simulink library "PTOSim_Lib_Updated"  (R2020b)
settings: Solver=ode45  StartTime=0.0  StopTime=10.0  RelTol=1e-3  EnableMultiTasking=on
undefined symbols (not defined in the file or in its folder): DiscIntNeverNeededParam, pAeq, pAupper_limit, pBeq, pBupper_limit, ptosim, table
libraries: simulink x2, $bdroot x1
(part 2 of 2)

== system PTOSim_Lib_Updated/Generator/Direct Drive Rotary Generator/Subsystem ==
  vsdq : Inport
  wd : Inport  Port=2
  Add : Sum  Inputs=+-+
  Add1 : Sum  Inputs=--+
  Demux2 : Demux  Outputs=2
      settings: DisplayOption=none
  Fcn : Fcn  Expr=( u(1) - ptosim.lambda_fd ) / ptosim.Ls
  Gain : Gain  Gain=1/ptosim.Ls
  Gain1 : Gain  Gain=(pi*ptosim.radius/ptosim.tau_p)*ptosim.lambda_fd
  Gain2 : Gain  Gain=ptosim.Rs
  Gain3 : Gain  Gain=ptosim.Rs
  Integrator : Integrator  InitialCondition=ptosim.lambda_sd_0
  Integrator1 : Integrator  InitialCondition=ptosim.lambda_sq_0
  Mux : Mux  Inputs=2
  Product : Product  RndMeth=Zero
  Product1 : Product  RndMeth=Zero
  Tem : Outport
  isdq : Outport  Port=2
  wires:
  Add/1 -> Integrator/1  "d_dt_lambda_sd"
  Integrator/1 -> Product1/2, Fcn/1  "lambda_sd"
  Fcn/1 -> Gain3/1, Mux/1  "isd"
  Product/1 -> Add/1
  Add1/1 -> Integrator1/1  "d_dt_lambda_sq"
  Integrator1/1 -> Gain/1, Product/2  "lambda_sq"
  wd/1 -> Product1/1, Product/1
  Gain/1 -> Gain2/1, Mux/2, Gain1/1  "isq"
  Product1/1 -> Add1/1
  Demux2/1 -> Add/3  "vsd"
  Demux2/2 -> Add1/3  "vsq"
  vsdq/1 -> Demux2/1  "vsdq"
  Gain3/1 -> Add/2  "isd_Rs"
  Gain2/1 -> Add1/2
  Mux/1 -> isdq/1  "isdq"
  Gain1/1 -> Tem/1

== system PTOSim_Lib_Updated/Hydraulic/Compressible Fluid Piston/Pressure Bottom ==
  pos : Inport
  volFlowBottom : Inport  Port=2
  volFLowP : Inport  Port=3
  Constant1 : Constant  Value=ptosim.Vo
  Divide1 : Product  Inputs=*/
  Gain4 : Gain  Gain=ptosim.Beta_e
  Gain5 : Gain  Gain=ptosim.Ap
  Integrator3 : Integrator  InitialCondition=ptosim.pBi  UpperSaturationLimit=pBupper_limit  LowerSaturationLimit=pBeq
  Sum2 : Sum  Inputs=+-
  Sum3 : Sum
  bottomPressure : Outport
  wires:
  volFLowP/1 -> Sum2/2
  Integrator3/1 -> bottomPressure/1
  volFlowBottom/1 -> Sum2/1
  Divide1/1 -> Integrator3/1
  Sum3/1 -> Divide1/2
  Gain4/1 -> Divide1/1
  Constant1/1 -> Sum3/2
  Gain5/1 -> Sum3/1
  pos/1 -> Gain5/1
  Sum2/1 -> Gain4/1

== system PTOSim_Lib_Updated/Hydraulic/Compressible Fluid Piston/Pressure Top ==
  pos : Inport
  volFlowTop : Inport  Port=2
  volFlowP : Inport  Port=3
  Constant : Constant  Value=ptosim.Vo
  Divide : Product  Inputs=*/
  Gain1 : Gain  Gain=ptosim.Beta_e
  Gain2 : Gain  Gain=ptosim.Ap
  Integrator2 : Integrator  InitialCondition=ptosim.pAi  UpperSaturationLimit=pAupper_limit  LowerSaturationLimit=pAeq
  Sum : Sum
  Sum1 : Sum  Inputs=-+
  topPressure : Outport
  wires:
  volFlowP/1 -> Sum/2
  Integrator2/1 -> topPressure/1
  Divide/1 -> Integrator2/1
  volFlowTop/1 -> Sum/1
  Sum1/1 -> Divide/2
  Gain1/1 -> Divide/1
  Constant/1 -> Sum1/2
  Gain2/1 -> Sum1/1
  pos/1 -> Gain2/1
  Sum/1 -> Gain1/1

== system PTOSim_Lib_Updated/Hydraulic/Compressible Fluid Piston Updated/Subsystem ==
  Pos : Inport
  Vel : Inport  Port=2
  QB : Inport  Port=3
  Add : Sum
  Add1 : Sum  Inputs=--+
  Constant : Constant  Value=ptosim.Ap_B
  Constant1 : Constant  Value=ptosim.PistonStroke
  Constant2 : Constant  Value=ptosim.Ap_B
  Constant3 : Constant  Value=ptosim.BulkModulus
  Constant4 : Constant  Value=ptosim.xi_piston
  Divide : Product  Inputs=/*
  Product : Product
  Product1 : Product
  Product2 : Product
  Saturation : Saturate  UpperLimit=inf  LowerLimit=1e-12
  dPB_dt : Outport
  wires:
  Constant4/1 -> Add1/2
  Constant1/1 -> Add1/3
  Product1/1 -> dPB_dt/1
  Divide/1 -> Product1/1
  Constant3/1 -> Divide/2
  Product2/1 -> Saturation/1
  Constant2/1 -> Product2/2
  Add1/1 -> Product2/1
  Pos/1 -> Add1/1
  Add/1 -> Product1/2
  QB/1 -> Add/2
  Product/1 -> Add/1
  Constant/1 -> Product/2
  Vel/1 -> Product/1
  Saturation/1 -> Divide/1

== system PTOSim_Lib_Updated/Hydraulic/Compressible Fluid Piston Updated/dPa_dt ==
  Pos : Inport
  Vel : Inport  Port=2
  QA : Inport  Port=3
  Add : Sum  Inputs=-+
  Add1 : Sum
  Constant : Constant  Value=ptosim.Ap_A
  Constant1 : Constant  Value=ptosim.BulkModulus/ptosim.Ap_A
  Constant2 : Constant  Value=ptosim.xi_piston
  Divide : Product  Inputs=/*
  Product : Product
  Product1 : Product
  Saturation : Saturate  UpperLimit=inf  LowerLimit=1e-12
  dPA_dt : Outport
  wires:
  Constant2/1 -> Add1/1
  Add1/1 -> Saturation/1
  Pos/1 -> Add1/2
  Product/1 -> Add/1
  QA/1 -> Add/2
  Constant/1 -> Product/2
  Add/1 -> Product1/2
  Divide/1 -> dPA_dt/1
  Constant1/1 -> Product1/1
  Product1/1 -> Divide/2
  Vel/1 -> Product/1
  Saturation/1 -> Divide/1

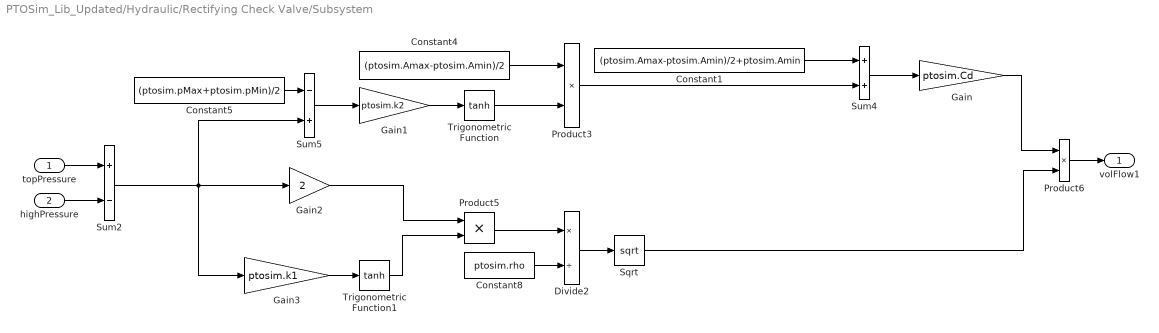
== system PTOSim_Lib_Updated/Hydraulic/Rectifying Check Valve/Subsystem ==
  topPressure : Inport
  highPressure : Inport  Port=2
  Constant1 : Constant  Value=(ptosim.Amax-ptosim.Amin)/2+ptosim.Amin
  Constant4 : Constant  Value=(ptosim.Amax-ptosim.Amin)/2
  Constant5 : Constant  Value=(ptosim.pMax+ptosim.pMin)/2
  Constant8 : Constant  Value=ptosim.rho
  Divide2 : Product  Inputs=*/
  Gain : Gain  Gain=ptosim.Cd
  Gain1 : Gain  Gain=ptosim.k2
  Gain2 : Gain  Gain=2
  Gain3 : Gain  Gain=ptosim.k1
  Product3 : Product
  Product5 : Product
  Product6 : Product
  Sqrt : Sqrt  SaturateOnIntegerOverflow=on
  Sum2 : Sum  Inputs=+-
  Sum4 : Sum
  Sum5 : Sum  Inputs=-+
  Trigonometric Function : Trigonometry  Operator=tanh
  Trigonometric Function1 : Trigonometry  Operator=tanh
  volFlow1 : Outport
  wires:
  Gain1/1 -> Trigonometric Function/1
  Trigonometric Function/1 -> Product3/2
  Product3/1 -> Sum4/2
  Sum5/1 -> Gain1/1
  Sum4/1 -> Gain/1
  Gain3/1 -> Trigonometric Function1/1
  Gain2/1 -> Product5/1
  Trigonometric Function1/1 -> Product5/2
  Sqrt/1 -> Product6/2
  Gain/1 -> Product6/1
  Constant8/1 -> Divide2/2
  Product5/1 -> Divide2/1
  Divide2/1 -> Sqrt/1
  topPressure/1 -> Sum2/1
  highPressure/1 -> Sum2/2
  Product6/1 -> volFlow1/1
  Constant4/1 -> Product3/1
  Constant5/1 -> Sum5/1
  Constant1/1 -> Sum4/1
  Sum2/1 -> Gain3/1, Sum5/2, Gain2/1

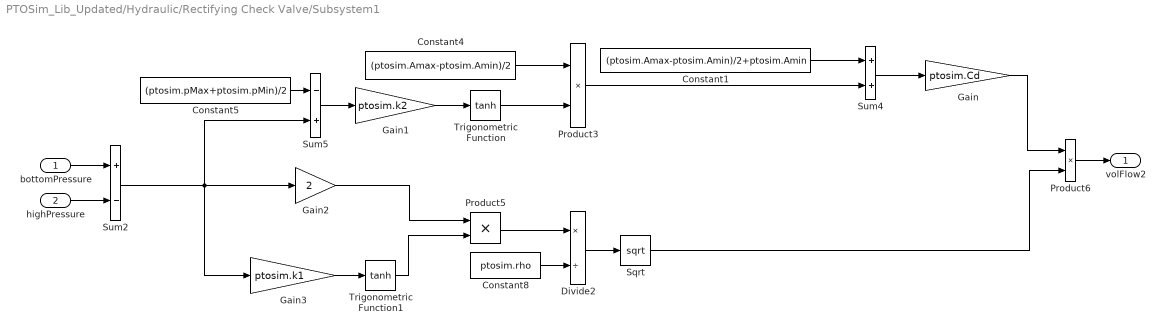
== system PTOSim_Lib_Updated/Hydraulic/Rectifying Check Valve/Subsystem1 ==
  bottomPressure : Inport
  highPressure : Inport  Port=2
  Constant1 : Constant  Value=(ptosim.Amax-ptosim.Amin)/2+ptosim.Amin
  Constant4 : Constant  Value=(ptosim.Amax-ptosim.Amin)/2
  Constant5 : Constant  Value=(ptosim.pMax+ptosim.pMin)/2
  Constant8 : Constant  Value=ptosim.rho
  Divide2 : Product  Inputs=*/
  Gain : Gain  Gain=ptosim.Cd
  Gain1 : Gain  Gain=ptosim.k2
  Gain2 : Gain  Gain=2
  Gain3 : Gain  Gain=ptosim.k1
  Product3 : Product
  Product5 : Product
  Product6 : Product
  Sqrt : Sqrt  SaturateOnIntegerOverflow=on
  Sum2 : Sum  Inputs=+-
  Sum4 : Sum
  Sum5 : Sum  Inputs=-+
  Trigonometric Function : Trigonometry  Operator=tanh
  Trigonometric Function1 : Trigonometry  Operator=tanh
  volFlow2 : Outport
  wires:
  Gain1/1 -> Trigonometric Function/1
  Trigonometric Function/1 -> Product3/2
  Product3/1 -> Sum4/2
  Sum5/1 -> Gain1/1
  Sum4/1 -> Gain/1
  Gain3/1 -> Trigonometric Function1/1
  Gain2/1 -> Product5/1
  Trigonometric Function1/1 -> Product5/2
  Sqrt/1 -> Product6/2
  Gain/1 -> Product6/1
  Constant8/1 -> Divide2/2
  Product5/1 -> Divide2/1
  Divide2/1 -> Sqrt/1
  bottomPressure/1 -> Sum2/1
  highPressure/1 -> Sum2/2
  Product6/1 -> volFlow2/1
  Constant4/1 -> Product3/1
  Constant5/1 -> Sum5/1
  Constant1/1 -> Sum4/1
  Sum2/1 -> Gain3/1, Sum5/2, Gain2/1

== system PTOSim_Lib_Updated/Hydraulic/Rectifying Check Valve/Subsystem2 ==
  lowPressure : Inport
  bottomPressure : Inport  Port=2
  Constant1 : Constant  Value=(ptosim.Amax-ptosim.Amin)/2+ptosim.Amin
  Constant4 : Constant  Value=(ptosim.Amax-ptosim.Amin)/2
  Constant5 : Constant  Value=(ptosim.pMax+ptosim.pMin)/2
  Constant8 : Constant  Value=ptosim.rho
  Divide2 : Product  Inputs=*/
  Gain : Gain  Gain=ptosim.Cd
  Gain1 : Gain  Gain=ptosim.k2
  Gain2 : Gain  Gain=2
  Gain3 : Gain  Gain=ptosim.k1
  Product3 : Product
  Product5 : Product
  Product6 : Product
  Sqrt : Sqrt  SaturateOnIntegerOverflow=on
  Sum2 : Sum  Inputs=+-
  Sum4 : Sum
  Sum5 : Sum  Inputs=-+
  Trigonometric Function : Trigonometry  Operator=tanh
  Trigonometric Function1 : Trigonometry  Operator=tanh
  volFlow3 : Outport
  wires:
  Gain1/1 -> Trigonometric Function/1
  Trigonometric Function/1 -> Product3/2
  Product3/1 -> Sum4/2
  Sum5/1 -> Gain1/1
  Sum4/1 -> Gain/1
  Gain3/1 -> Trigonometric Function1/1
  Gain2/1 -> Product5/1
  Trigonometric Function1/1 -> Product5/2
  Sqrt/1 -> Product6/2
  Gain/1 -> Product6/1
  Constant8/1 -> Divide2/2
  Product5/1 -> Divide2/1
  Divide2/1 -> Sqrt/1
  lowPressure/1 -> Sum2/1
  bottomPressure/1 -> Sum2/2
  Product6/1 -> volFlow3/1
  Constant4/1 -> Product3/1
  Constant5/1 -> Sum5/1
  Constant1/1 -> Sum4/1
  Sum2/1 -> Gain3/1, Sum5/2, Gain2/1

== system PTOSim_Lib_Updated/Hydraulic/Rectifying Check Valve/Subsystem3 ==
  lowPressure : Inport
  topPressure : Inport  Port=2
  Constant1 : Constant  Value=(ptosim.Amax-ptosim.Amin)/2+ptosim.Amin
  Constant4 : Constant  Value=(ptosim.Amax-ptosim.Amin)/2
  Constant5 : Constant  Value=(ptosim.pMax+ptosim.pMin)/2
  Constant8 : Constant  Value=ptosim.rho
  Divide2 : Product  Inputs=*/
  Gain : Gain  Gain=ptosim.Cd
  Gain1 : Gain  Gain=ptosim.k2
  Gain2 : Gain  Gain=2
  Gain3 : Gain  Gain=ptosim.k1
  Product3 : Product
  Product5 : Product
  Product6 : Product
  Sqrt : Sqrt  SaturateOnIntegerOverflow=on
  Sum2 : Sum  Inputs=+-
  Sum4 : Sum
  Sum5 : Sum  Inputs=-+
  Trigonometric Function : Trigonometry  Operator=tanh
  Trigonometric Function1 : Trigonometry  Operator=tanh
  volFlow4 : Outport
  wires:
  Gain1/1 -> Trigonometric Function/1
  Trigonometric Function/1 -> Product3/2
  Product3/1 -> Sum4/2
  Sum5/1 -> Gain1/1
  Sum4/1 -> Gain/1
  Gain3/1 -> Trigonometric Function1/1
  Gain2/1 -> Product5/1
  Trigonometric Function1/1 -> Product5/2
  Sqrt/1 -> Product6/2
  Gain/1 -> Product6/1
  Constant8/1 -> Divide2/2
  Product5/1 -> Divide2/1
  Divide2/1 -> Sqrt/1
  lowPressure/1 -> Sum2/1
  topPressure/1 -> Sum2/2
  Product6/1 -> volFlow4/1
  Constant4/1 -> Product3/1
  Constant5/1 -> Sum5/1
  Constant1/1 -> Sum4/1
  Sum2/1 -> Gain3/1, Sum5/2, Gain2/1

== system PTOSim_Lib_Updated/Motion Conversion/Rotary to Linear Adjustable Rod/Angle Calculation for PTO ==
  angPos : Inport
  Add : Sum  Inputs=+-
  Add1 : Sum  Inputs=+-
  Constant1 : Constant  Value=ptosim.crank
  Constant2 : Constant  Value=ptosim.crank
  Constant3 : Constant  Value=ptosim.offset
  Distance btw flap joint & rod joint along x-axis : $bdroot/Motion Conversion/Rotary to Linear Adjustable Rod/Angular to Linear Velocity/Subsystem/Distance btw flap joint & rod joint along x-axis  SystemSampleTime=-1  VariantActivationTime=update diagram  Latency=0  AutoFrameSizeCalculation=off
  Divide : Product  Inputs=*/
  Divide1 : Product  Inputs=*/
  Product : Product
  Product1 : Product
  Subsystem1 : Subsystem  AncestorBlock=|
      | PTOSim_Lib/Motion Conversion/Rotary to Linear
      | Adjustable Rod/Angular to Linear
      | Velocity/Subsystem
  Subsystem2 : Subsystem  AncestorBlock=|
      | PTOSim_Lib/Motion Conversion/Rotary to Linear
      | Adjustable Rod/Angular to Linear
      | Velocity/Subsystem
  Trigonometric Function : Trigonometry
  Trigonometric Function1 : Trigonometry  Operator=cos
  Cos_gamma : Outport
  Sin_gamma : Outport  Port=2
  wires:
  Trigonometric Function/1 -> Product/1
  Product/1 -> Add/1
  Distance btw flap joint & rod joint along x-axis/1 -> Add/2
  Constant2/1 -> Product/2
  Add/1 -> Divide/1
  Subsystem1/1(rodLength) -> Divide/2
  Divide/1 -> Cos_gamma/1
  Subsystem2/1(rodLength) -> Divide1/2
  Trigonometric Function1/1 -> Product1/1
  Constant1/1 -> Product1/2
  Product1/1 -> Add1/1
  Constant3/1 -> Add1/2
  Add1/1 -> Divide1/1
  angPos/1 -> Subsystem1/1(angPos), Subsystem2/1(angPos), Trigonometric Function1/1, Trigonometric Function/1
  Divide1/1 -> Sin_gamma/1

== system PTOSim_Lib_Updated/Motion Conversion/Rotary to Linear Adjustable Rod/Angular to Linear Position ==
  angPos : Inport
  Add1 : Sum  Inputs=+-
  Add2 : Sum  Inputs=+-
  Add5 : Sum
  Add6 : Sum  Inputs=+-
  Constant1 : Constant  Value=ptosim.rodInit
  Constant2 : Constant  Value=ptosim.crank
  Constant3 : Constant  Value=ptosim.offset
  Constant7 : Constant  Value=ptosim.crank
  Distance btw flap joint & rod joint along x-axis : Subsystem
  Math Function1 : Math  Operator=square  SignedPower=on  SaturateOnIntegerOverflow=on
  Math Function6 : Math  Operator=square  SignedPower=on  SaturateOnIntegerOverflow=on
  Product1 : Product  Inputs=**
  Product7 : Product  Inputs=**
  Sqrt2 : Sqrt  SaturateOnIntegerOverflow=on
  Trigonometric Function1 : Trigonometry  Operator=cos
  Trigonometric Function5 : Trigonometry
  linearPos : Outport
  wires:
  angPos/1 -> Trigonometric Function5/1, Trigonometric Function1/1
  Add1/1 -> linearPos/1
  Add2/1 -> Math Function1/1
  Trigonometric Function5/1 -> Product7/2
  Product7/1 -> Add6/2
  Add6/1 -> Math Function6/1
  Math Function6/1 -> Add5/2
  Add5/1 -> Sqrt2/1
  Sqrt2/1 -> Add1/2
  Constant1/1 -> Add1/1
  Constant2/1 -> Product1/1
  Trigonometric Function1/1 -> Product1/2
  Product1/1 -> Add2/1
  Constant3/1 -> Add2/2
  Math Function1/1 -> Add5/1
  Constant7/1 -> Product7/1
  Distance btw flap joint & rod joint along x-axis/1(d) -> Add6/1

== system PTOSim_Lib_Updated/Motion Conversion/Rotary to Linear Adjustable Rod/Angular to Linear Velocity ==
  angPos : Inport
  angVel : Inport  Port=2
  Add1 : Sum  Inputs=+-
  Add2 : Sum  Inputs=+-
  Add3 : Sum  Inputs=-+
  Constant1 : Constant  Value=ptosim.crank
  Constant2 : Constant  Value=ptosim.crank
  Constant3 : Constant  Value=ptosim.offset
  Constant7 : Constant  Value=ptosim.crank
  Distance btw flap joint & rod joint along x-axis : Subsystem
  Divide1 : Product  Inputs=*/
  Product1 : Product  Inputs=**
  Product2 : Product  Inputs=***
  Product3 : Product  Inputs=**
  Product4 : Product  Inputs=***
  Product7 : Product  Inputs=**
  Subsystem : Subsystem
  Trigonometric Function1 : Trigonometry  Operator=cos
  Trigonometric Function2 : Trigonometry  Operator=cos
  Trigonometric Function5 : Trigonometry
  linearVel : Outport
  wires:
  Add2/1 -> Product2/1
  Constant2/1 -> Product1/1
  Trigonometric Function1/1 -> Product1/2
  Product1/1 -> Add2/1
  Constant3/1 -> Add2/2
  Trigonometric Function5/1 -> Product7/2
  Product7/1 -> Add1/1, Product2/2
  Constant7/1 -> Product7/1
  angVel/1 -> Product2/3, Product4/1
  Distance btw flap joint & rod joint along x-axis/1(d) -> Add1/2
  Constant1/1 -> Product3/1
  Trigonometric Function2/1 -> Product3/2
  Product3/1 -> Product4/3
  angPos/1 -> Trigonometric Function5/1, Trigonometric Function2/1, Trigonometric Function1/1, Subsystem/1(angPos)
  Add1/1 -> Product4/2
  Subsystem/1(rodLength) -> Divide1/2
  Product2/1 -> Add3/1
  Product4/1 -> Add3/2
  Add3/1 -> Divide1/1
  Divide1/1 -> linearVel/1

== system PTOSim_Lib_Updated/Motion Conversion/Rotary to Linear Crank/Angular to Linear Position ==
  angPos : Inport
  Add1 : Sum  Inputs=++-
  Add2 : Sum  Inputs=+-
  Add5 : Sum  Inputs=+-
  Constant1 : Constant  Value=ptosim.rodLength
  Constant2 : Constant  Value=ptosim.crank
  Constant3 : Constant  Value=ptosim.offset
  Constant7 : Constant  Value=ptosim.crank
  Initial Distance btw flap joint & crank joint along x-axis : Subsystem
  Math Function1 : Math  Operator=square  SignedPower=on  SaturateOnIntegerOverflow=on
  Math Function2 : Math  Operator=square  SignedPower=on  SaturateOnIntegerOverflow=on
  Product1 : Product  Inputs=**
  Product7 : Product  Inputs=**
  Sqrt2 : Sqrt  SaturateOnIntegerOverflow=on
  Trigonometric Function1 : Trigonometry  Operator=cos
  Trigonometric Function5 : Trigonometry
  linearPos : Outport
  wires:
  angPos/1 -> Trigonometric Function1/1, Trigonometric Function5/1
  Add2/1 -> Math Function1/1
  Trigonometric Function5/1 -> Product7/2
  Add5/1 -> Sqrt2/1
  Constant2/1 -> Product1/1
  Trigonometric Function1/1 -> Product1/2
  Product1/1 -> Add2/1
  Constant3/1 -> Add2/2
  Constant7/1 -> Product7/1
  Initial Distance btw flap joint & crank joint along x-axis/1(d) -> Add1/3
  Constant1/1 -> Math Function2/1
  Math Function1/1 -> Add5/2
  Sqrt2/1 -> Add1/2
  Product7/1 -> Add1/1
  Add1/1 -> linearPos/1
  Math Function2/1 -> Add5/1

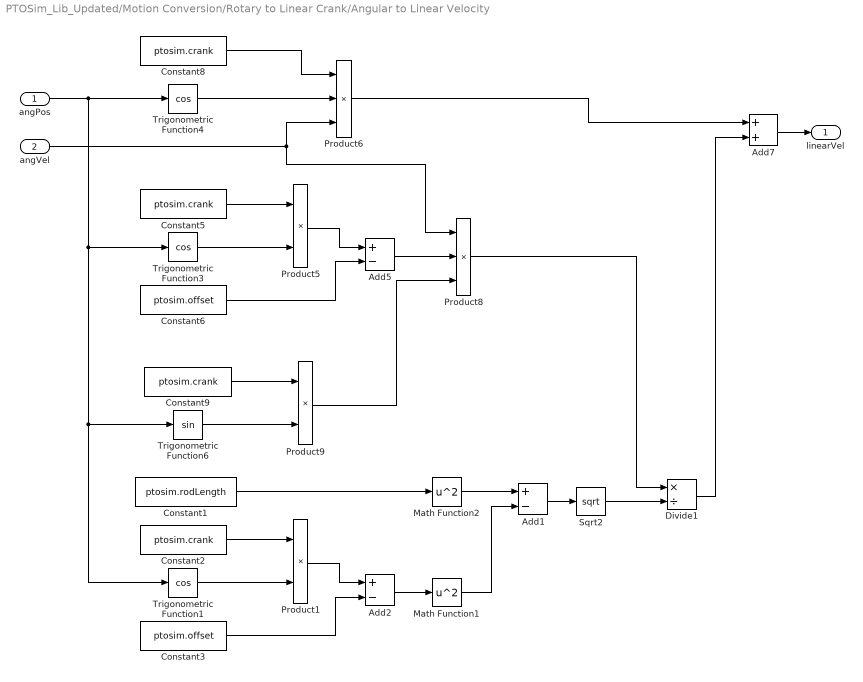
== system PTOSim_Lib_Updated/Motion Conversion/Rotary to Linear Crank/Angular to Linear Velocity ==
  angPos : Inport
  angVel : Inport  Port=2
  Add1 : Sum  Inputs=+-
  Add2 : Sum  Inputs=+-
  Add5 : Sum  Inputs=+-
  Add7 : Sum
  Constant1 : Constant  Value=ptosim.rodLength
  Constant{2,5,8..9} (4 alike) : Constant  Value=ptosim.crank
  Constant3 : Constant  Value=ptosim.offset
  Constant6 : Constant  Value=ptosim.offset
  Divide1 : Product  Inputs=*/
  Math Function1 : Math  Operator=square  SignedPower=on  SaturateOnIntegerOverflow=on
  Math Function2 : Math  Operator=square  SignedPower=on  SaturateOnIntegerOverflow=on
  Product1 : Product  Inputs=**
  Product5 : Product  Inputs=**
  Product6 : Product  Inputs=***
  Product8 : Product  Inputs=***
  Product9 : Product  Inputs=**
  Sqrt2 : Sqrt  SaturateOnIntegerOverflow=on
  Trigonometric Function1 : Trigonometry  Operator=cos
  Trigonometric Function3 : Trigonometry  Operator=cos
  Trigonometric Function4 : Trigonometry  Operator=cos
  Trigonometric Function6 : Trigonometry
  linearVel : Outport
  wires:
  Add7/1 -> linearVel/1
  Trigonometric Function4/1 -> Product6/2
  Constant8/1 -> Product6/1
  Product6/1 -> Add7/1
  Constant5/1 -> Product5/1
  Trigonometric Function3/1 -> Product5/2
  Product5/1 -> Add5/1
  Constant6/1 -> Add5/2
  Constant9/1 -> Product9/1
  Trigonometric Function6/1 -> Product9/2
  angVel/1 -> Product8/1, Product6/3
  Add5/1 -> Product8/2
  Product9/1 -> Product8/3
  angPos/1 -> Trigonometric Function1/1, Trigonometric Function6/1, Trigonometric Function3/1, Trigonometric Function4/1
  Add2/1 -> Math Function1/1
  Add1/1 -> Sqrt2/1
  Constant2/1 -> Product1/1
  Trigonometric Function1/1 -> Product1/2
  Product1/1 -> Add2/1
  Constant3/1 -> Add2/2
  Constant1/1 -> Math Function2/1
  Math Function1/1 -> Add1/2
  Sqrt2/1 -> Divide1/2
  Product8/1 -> Divide1/1
  Divide1/1 -> Add7/2
  Math Function2/1 -> Add1/1

== system PTOSim_Lib_Updated/Motion Conversion/Rotary to Linear Crank/Subsystem ==
  angle : Inport
  Add : Sum  Inputs=+-
  Add1 : Sum  Inputs=+-
  Constant : Constant
  Constant2 : Constant  Value=ptosim.crank
  Constant3 : Constant  Value=ptosim.offset
  Constant4 : Constant  Value=ptosim.rodLength
  Divide : Product  Inputs=*/
  Product : Product
  Sqrt : Sqrt  SaturateOnIntegerOverflow=on
  Square : Math  Operator=square  SignedPower=on  SaturateOnIntegerOverflow=on
  Trigonometric Function : Trigonometry  Operator=cos
  abs(cos_gamma) : Outport
  wires:
  angle/1 -> Trigonometric Function/1
  Trigonometric Function/1 -> Product/1
  Constant2/1 -> Product/2
  Product/1 -> Add/1
  Constant3/1 -> Add/2
  Add/1 -> Divide/1
  Constant4/1 -> Divide/2
  Divide/1 -> Square/1
  Square/1 -> Add1/2
  Add1/1 -> Sqrt/1
  Constant/1 -> Add1/1
  Sqrt/1 -> abs(cos_gamma)/1

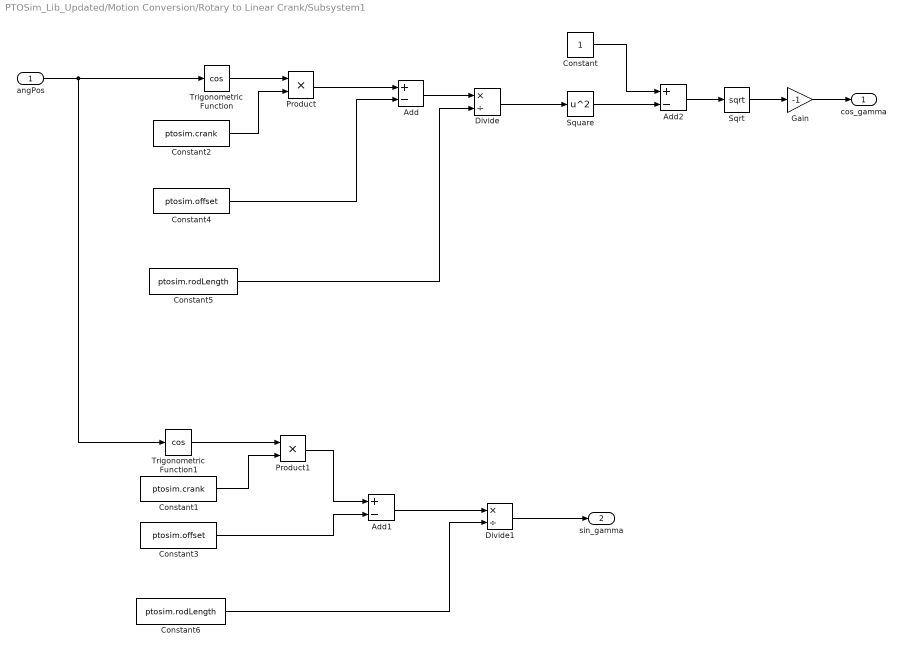
== system PTOSim_Lib_Updated/Motion Conversion/Rotary to Linear Crank/Subsystem1 ==
  angPos : Inport
  Add : Sum  Inputs=+-
  Add1 : Sum  Inputs=+-
  Add2 : Sum  Inputs=+-
  Constant : Constant
  Constant1 : Constant  Value=ptosim.crank
  Constant2 : Constant  Value=ptosim.crank
  Constant3 : Constant  Value=ptosim.offset
  Constant4 : Constant  Value=ptosim.offset
  Constant5 : Constant  Value=ptosim.rodLength
  Constant6 : Constant  Value=ptosim.rodLength
  Divide : Product  Inputs=*/
  Divide1 : Product  Inputs=*/
  Gain : Gain  Gain=-1
  Product : Product
  Product1 : Product
  Sqrt : Sqrt  SaturateOnIntegerOverflow=on
  Square : Math  Operator=square  SignedPower=on  SaturateOnIntegerOverflow=on
  Trigonometric Function : Trigonometry  Operator=cos
  Trigonometric Function1 : Trigonometry  Operator=cos
  cos_gamma : Outport
  sin_gamma : Outport  Port=2
  wires:
  Divide1/1 -> sin_gamma/1
  Add1/1 -> Divide1/1
  Constant3/1 -> Add1/2
  Product1/1 -> Add1/1
  Constant1/1 -> Product1/2
  Trigonometric Function1/1 -> Product1/1
  Constant6/1 -> Divide1/2
  Add/1 -> Divide/1
  Add2/1 -> Sqrt/1
  angPos/1 -> Trigonometric Function1/1, Trigonometric Function/1
  Square/1 -> Add2/2
  Product/1 -> Add/1
  Constant2/1 -> Product/2
  Trigonometric Function/1 -> Product/1
  Divide/1 -> Square/1
  Constant5/1 -> Divide/2
  Constant/1 -> Add2/1
  Constant4/1 -> Add/2
  Sqrt/1 -> Gain/1
  Gain/1 -> cos_gamma/1

== system PTOSim_Lib_Updated/Motion Conversion/Rotary to Linear Adjustable Rod/Angle Calculation for PTO/Subsystem1 ==
  angPos : Inport
  Add2 : Sum  Inputs=+-
  Add5 : Sum
  Add6 : Sum  Inputs=+-
  Constant1 : Constant  Value=ptosim.crank
  Constant2 : Constant  Value=ptosim.crank
  Constant3 : Constant  Value=ptosim.offset
  Distance btw flap joint & rod joint along x-axis : Subsystem
  Math Function1 : Math  Operator=square  SignedPower=on  SaturateOnIntegerOverflow=on
  Math Function6 : Math  Operator=square  SignedPower=on  SaturateOnIntegerOverflow=on
  Product1 : Product  Inputs=**
  Product7 : Product  Inputs=**
  Sqrt2 : Sqrt  SaturateOnIntegerOverflow=on
  Trigonometric Function1 : Trigonometry  Operator=cos
  Trigonometric Function5 : Trigonometry
  rodLength : Outport
  wires:
  Distance btw flap joint & rod joint along x-axis/1(d) -> Add6/1
  Constant2/1 -> Product7/1
  Math Function1/1 -> Add5/1
  Constant3/1 -> Add2/2
  Product1/1 -> Add2/1
  Trigonometric Function1/1 -> Product1/2
  Constant1/1 -> Product1/1
  Sqrt2/1 -> rodLength/1
  Add5/1 -> Sqrt2/1
  Math Function6/1 -> Add5/2
  Add6/1 -> Math Function6/1
  Product7/1 -> Add6/2
  Trigonometric Function5/1 -> Product7/2
  Add2/1 -> Math Function1/1
  angPos/1 -> Trigonometric Function1/1, Trigonometric Function5/1

== system PTOSim_Lib_Updated/Motion Conversion/Rotary to Linear Adjustable Rod/Angle Calculation for PTO/Subsystem2 ==
  angPos : Inport
  Add2 : Sum  Inputs=+-
  Add5 : Sum
  Add6 : Sum  Inputs=+-
  Constant1 : Constant  Value=ptosim.crank
  Constant2 : Constant  Value=ptosim.crank
  Constant3 : Constant  Value=ptosim.offset
  Distance btw flap joint & rod joint along x-axis : Subsystem
  Math Function1 : Math  Operator=square  SignedPower=on  SaturateOnIntegerOverflow=on
  Math Function6 : Math  Operator=square  SignedPower=on  SaturateOnIntegerOverflow=on
  Product1 : Product  Inputs=**
  Product7 : Product  Inputs=**
  Sqrt2 : Sqrt  SaturateOnIntegerOverflow=on
  Trigonometric Function1 : Trigonometry  Operator=cos
  Trigonometric Function5 : Trigonometry
  rodLength : Outport
  wires:
  Distance btw flap joint & rod joint along x-axis/1(d) -> Add6/1
  Constant2/1 -> Product7/1
  Math Function1/1 -> Add5/1
  Constant3/1 -> Add2/2
  Product1/1 -> Add2/1
  Trigonometric Function1/1 -> Product1/2
  Constant1/1 -> Product1/1
  Sqrt2/1 -> rodLength/1
  Add5/1 -> Sqrt2/1
  Math Function6/1 -> Add5/2
  Add6/1 -> Math Function6/1
  Product7/1 -> Add6/2
  Trigonometric Function5/1 -> Product7/2
  Add2/1 -> Math Function1/1
  angPos/1 -> Trigonometric Function1/1, Trigonometric Function5/1

== system PTOSim_Lib_Updated/Motion Conversion/Rotary to Linear Adjustable Rod/Angular to Linear Position/Distance btw flap joint & rod joint along x-axis ==
  Add3 : Sum  Inputs=+-
  Add4 : Sum  Inputs=+-
  Constant4 : Constant  Value=ptosim.rodInit
  Constant5 : Constant  Value=ptosim.crank
  Constant6 : Constant  Value=ptosim.offset
  Math Function2 : Math  Operator=square  SignedPower=on  SaturateOnIntegerOverflow=on
  Math Function3 : Math  Operator=square  SignedPower=on  SaturateOnIntegerOverflow=on
  Sqrt1 : Sqrt  SaturateOnIntegerOverflow=on
  d : Outport
  wires:
  Add3/1 -> Sqrt1/1
  Constant4/1 -> Math Function2/1
  Constant5/1 -> Add4/1
  Constant6/1 -> Add4/2
  Add4/1 -> Math Function3/1
  Math Function3/1 -> Add3/2
  Math Function2/1 -> Add3/1
  Sqrt1/1 -> d/1

== system PTOSim_Lib_Updated/Motion Conversion/Rotary to Linear Adjustable Rod/Angular to Linear Velocity/Distance btw flap joint & rod joint along x-axis ==
  Add3 : Sum  Inputs=+-
  Add4 : Sum  Inputs=+-
  Constant4 : Constant  Value=ptosim.rodInit
  Constant5 : Constant  Value=ptosim.crank
  Constant6 : Constant  Value=ptosim.offset
  Math Function2 : Math  Operator=square  SignedPower=on  SaturateOnIntegerOverflow=on
  Math Function3 : Math  Operator=square  SignedPower=on  SaturateOnIntegerOverflow=on
  Sqrt1 : Sqrt  SaturateOnIntegerOverflow=on
  d : Outport
  wires:
  Add3/1 -> Sqrt1/1
  Constant4/1 -> Math Function2/1
  Constant5/1 -> Add4/1
  Constant6/1 -> Add4/2
  Add4/1 -> Math Function3/1
  Math Function3/1 -> Add3/2
  Math Function2/1 -> Add3/1
  Sqrt1/1 -> d/1

== system PTOSim_Lib_Updated/Motion Conversion/Rotary to Linear Adjustable Rod/Angular to Linear Velocity/Subsystem ==
  angPos : Inport
  Add2 : Sum  Inputs=+-
  Add5 : Sum
  Add6 : Sum  Inputs=+-
  Constant2 : Constant  Value=ptosim.crank
  Constant3 : Constant  Value=ptosim.offset
  Constant7 : Constant  Value=ptosim.crank
  Distance btw flap joint & rod joint along x-axis : Subsystem
  Math Function1 : Math  Operator=square  SignedPower=on  SaturateOnIntegerOverflow=on
  Math Function6 : Math  Operator=square  SignedPower=on  SaturateOnIntegerOverflow=on
  Product1 : Product  Inputs=**
  Product7 : Product  Inputs=**
  Sqrt2 : Sqrt  SaturateOnIntegerOverflow=on
  Trigonometric Function1 : Trigonometry  Operator=cos
  Trigonometric Function5 : Trigonometry
  rodLength : Outport
  wires:
  angPos/1 -> Trigonometric Function5/1, Trigonometric Function1/1
  Add2/1 -> Math Function1/1
  Trigonometric Function5/1 -> Product7/2
  Product7/1 -> Add6/2
  Add6/1 -> Math Function6/1
  Math Function6/1 -> Add5/2
  Add5/1 -> Sqrt2/1
  Sqrt2/1 -> rodLength/1
  Constant2/1 -> Product1/1
  Trigonometric Function1/1 -> Product1/2
  Product1/1 -> Add2/1
  Constant3/1 -> Add2/2
  Math Function1/1 -> Add5/1
  Constant7/1 -> Product7/1
  Distance btw flap joint & rod joint along x-axis/1(d) -> Add6/1

== system PTOSim_Lib_Updated/Motion Conversion/Rotary to Linear Crank/Angular to Linear Position/Initial Distance btw flap joint & crank joint along x-axis ==
  Add3 : Sum  Inputs=+-
  Add4 : Sum  Inputs=+-
  Constant1 : Constant  Value=ptosim.rodLength
  Constant5 : Constant  Value=ptosim.crank
  Constant6 : Constant  Value=ptosim.offset
  Math Function2 : Math  Operator=square  SignedPower=on  SaturateOnIntegerOverflow=on
  Math Function3 : Math  Operator=square  SignedPower=on  SaturateOnIntegerOverflow=on
  Sqrt1 : Sqrt  SaturateOnIntegerOverflow=on
  d : Outport
  wires:
  Add3/1 -> Sqrt1/1
  Constant1/1 -> Math Function2/1
  Constant5/1 -> Add4/1
  Constant6/1 -> Add4/2
  Add4/1 -> Math Function3/1
  Math Function3/1 -> Add3/2
  Math Function2/1 -> Add3/1
  Sqrt1/1 -> d/1

== system PTOSim_Lib_Updated/Motion Conversion/Rotary to Linear Adjustable Rod/Angle Calculation for PTO/Subsystem1/Distance btw flap joint & rod joint along x-axis ==
  Add3 : Sum  Inputs=+-
  Add4 : Sum  Inputs=+-
  Constant1 : Constant  Value=ptosim.crank
  Constant2 : Constant  Value=ptosim.rodInit
  Constant3 : Constant  Value=ptosim.offset
  Math Function2 : Math  Operator=square  SignedPower=on  SaturateOnIntegerOverflow=on
  Math Function3 : Math  Operator=square  SignedPower=on  SaturateOnIntegerOverflow=on
  Sqrt1 : Sqrt  SaturateOnIntegerOverflow=on
  d : Outport
  wires:
  Sqrt1/1 -> d/1
  Math Function2/1 -> Add3/1
  Math Function3/1 -> Add3/2
  Add4/1 -> Math Function3/1
  Constant3/1 -> Add4/2
  Constant1/1 -> Add4/1
  Constant2/1 -> Math Function2/1
  Add3/1 -> Sqrt1/1

== system PTOSim_Lib_Updated/Motion Conversion/Rotary to Linear Adjustable Rod/Angle Calculation for PTO/Subsystem2/Distance btw flap joint & rod joint along x-axis ==
  Add3 : Sum  Inputs=+-
  Add4 : Sum  Inputs=+-
  Constant1 : Constant  Value=ptosim.crank
  Constant2 : Constant  Value=ptosim.rodInit
  Constant3 : Constant  Value=ptosim.offset
  Math Function2 : Math  Operator=square  SignedPower=on  SaturateOnIntegerOverflow=on
  Math Function3 : Math  Operator=square  SignedPower=on  SaturateOnIntegerOverflow=on
  Sqrt1 : Sqrt  SaturateOnIntegerOverflow=on
  d : Outport
  wires:
  Sqrt1/1 -> d/1
  Math Function2/1 -> Add3/1
  Math Function3/1 -> Add3/2
  Add4/1 -> Math Function3/1
  Constant3/1 -> Add4/2
  Constant1/1 -> Add4/1
  Constant2/1 -> Math Function2/1
  Add3/1 -> Sqrt1/1

== system PTOSim_Lib_Updated/Motion Conversion/Rotary to Linear Adjustable Rod/Angular to Linear Velocity/Subsystem/Distance btw flap joint & rod joint along x-axis ==
  Add3 : Sum  Inputs=+-
  Add4 : Sum  Inputs=+-
  Constant4 : Constant  Value=ptosim.rodInit
  Constant5 : Constant  Value=ptosim.crank
  Constant6 : Constant  Value=ptosim.offset
  Math Function2 : Math  Operator=square  SignedPower=on  SaturateOnIntegerOverflow=on
  Math Function3 : Math  Operator=square  SignedPower=on  SaturateOnIntegerOverflow=on
  Sqrt1 : Sqrt  SaturateOnIntegerOverflow=on
  d : Outport
  wires:
  Add3/1 -> Sqrt1/1
  Constant4/1 -> Math Function2/1
  Constant5/1 -> Add4/1
  Constant6/1 -> Add4/2
  Add4/1 -> Math Function3/1
  Math Function3/1 -> Add3/2
  Math Function2/1 -> Add3/1
  Sqrt1/1 -> d/1
